simulink model "poster2"  (R2022a)
settings: Solver=VariableStepAuto  StartTime=0.0  StopTime=10.0  RelTol=1e-3
settings Model: Creator=feyzi  LastModifiedBy=feyzi

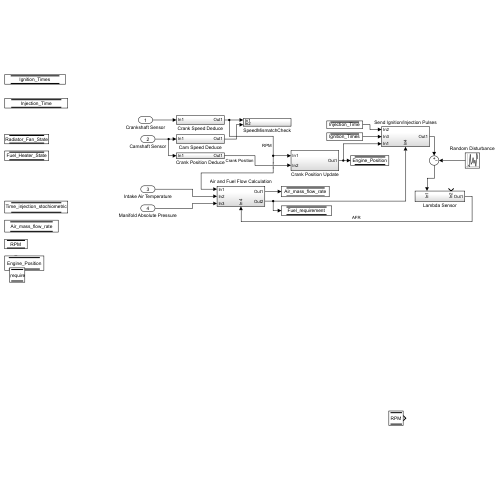
[thumbnail: Simulink's stored preview of the top-level diagram]
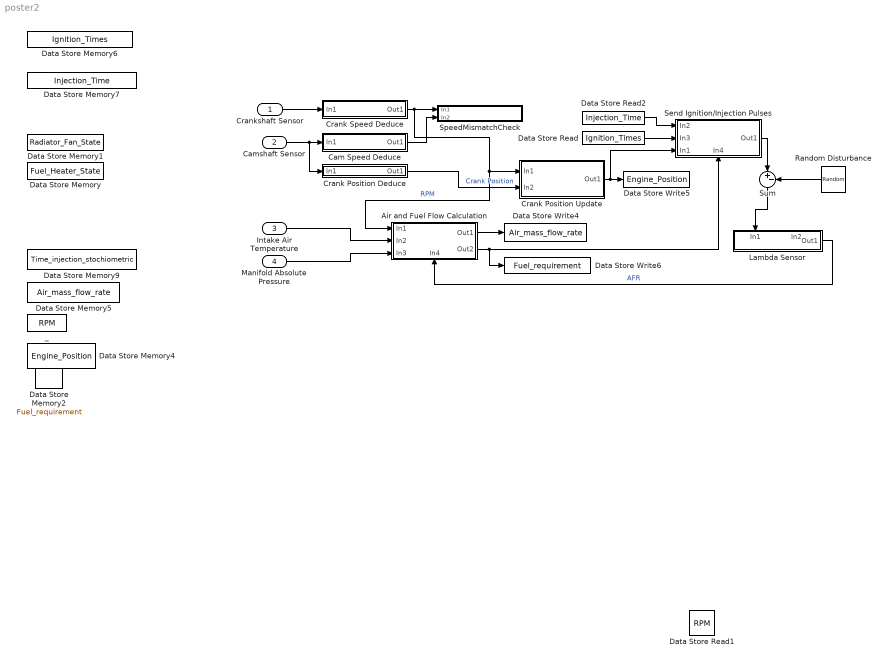
== system poster2 ==
  Crankshaft Sensor : Inport
  Camshaft Sensor : Inport  Port=2
  Intake Air Temperature : Inport  Port=3
  Manifold Absolute Pressure : Inport  Port=4
  Air and Fuel Flow Calculation : Subsystem
      settings: PortSchema="{\"entries\":[{\"content\":{\"sides\":[{\"content\":{\"connectorIds\":[\"In1\",\"In2\",\"In3\"]},\"type\":\"ConnectorPlacement.EquallySpacedRectSide\",\"uuid\":\"1a80d675-76df-4a65-b0a2-1f1f980be6c0\"},{\"content\":{\"connectorIds\":[\"Out1\",\"Out2\"],\"side\":\"RIGHT\"},\"type\":\"ConnectorPlacement.EquallySpacedRectSide\",\"uuid\":\"8955b592-f731-49d0-95be-21f996fa39e2\"},{\"content\":{\"connectorIds\":[],\"side\":\"TOP\"},\"type\":\"ConnectorPlacement.EquallySpacedRectSide\",\"uuid\":\"17a49bf9-f9ef-40a2-97c4-5293cd0c2b79\"},{\"content\":{\"connectorIds\":[\"In4\"],\"side\":\"BOTTOM\"},\"type\":\"ConnectorPlacement.EquallySpacedRectSide\",\"uuid\":\"0b8d33c3-a573-49dc-98b4-2c523fb61e9a\"}]},\"type\":\"ConnectorPlacement.EquallySpacedConnector\",\"uuid\":\"260580cd-7983-4c41-a340-dd72d4798db4\"}],\"packageUris\":[\"http://schema.mathworks.com/mf0/Connector/R2020b\"],\"version\":\"1.0\"}"
  Cam Speed Deduce : Subsystem
  Crank Position Deduce : Subsystem
  Crank Position Update : Subsystem
  Crank Speed Deduce : Subsystem
  Data Store Memory : DataStoreMemory  DataStoreName=Fuel_Heater_State  WriteAfterWriteMsg=warning  ShowAdditionalParam=off
  Data Store Memory1 : DataStoreMemory  DataStoreName=Radiator_Fan_State  WriteAfterWriteMsg=warning  ShowAdditionalParam=off
  Data Store Memory2 : DataStoreMemory  DataStoreName=Fuel_requirement  WriteAfterWriteMsg=warning  ShowAdditionalParam=off
  Data Store Memory4 : DataStoreMemory  DataStoreName=Engine_Position  WriteAfterWriteMsg=warning  ShowAdditionalParam=off
  Data Store Memory5 : DataStoreMemory  DataStoreName=Air_mass_flow_rate  WriteAfterWriteMsg=warning  ShowAdditionalParam=off
  Data Store Memory6 : DataStoreMemory  DataStoreName=Ignition_Times  WriteAfterWriteMsg=warning  ShowAdditionalParam=off
  Data Store Memory7 : DataStoreMemory  DataStoreName=Injection_Time  WriteAfterWriteMsg=warning  ShowAdditionalParam=off
  Data Store Memory9 : DataStoreMemory  DataStoreName=Time_injection_stochiometric  WriteAfterWriteMsg=warning  ShowAdditionalParam=off
  Data Store Read : DataStoreRead  DataStoreName=Ignition_Times  IndexOptions=Index vector (dialog)  Indices=1  OutputSizes=1
  Data Store Read1 : DataStoreRead  DataStoreName=RPM  IndexOptions=Index vector (dialog)  Indices=1  OutputSizes=1
  Data Store Read2 : DataStoreRead  DataStoreName=Injection_Time  IndexOptions=Index vector (dialog)  Indices=1  OutputSizes=1
  Data Store Write4 : DataStoreWrite  DataStoreName=Air_mass_flow_rate  IndexOptions=Index vector (dialog)  Indices=1  OutputSizes=1
  Data Store Write5 : DataStoreWrite  DataStoreName=Engine_Position  IndexOptions=Index vector (dialog)  Indices=1  OutputSizes=1
  Data Store Write6 : DataStoreWrite  DataStoreName=Fuel_requirement  IndexOptions=Index vector (dialog)  Indices=1  OutputSizes=1
  Lambda Sensor : Subsystem
      settings: PortSchema="{\"entries\":[{\"content\":{\"sides\":[{\"content\":{\"connectorIds\":[]},\"type\":\"ConnectorPlacement.EquallySpacedRectSide\",\"uuid\":\"be7673b4-920b-4ebb-aa7f-ea6b5173dfc7\"},{\"content\":{\"connectorIds\":[\"Out1\"],\"side\":\"RIGHT\"},\"type\":\"ConnectorPlacement.EquallySpacedRectSide\",\"uuid\":\"a4fdee98-027b-48e3-870e-bdd43bb26549\"},{\"content\":{\"connectorIds\":[\"In1\",\"In2\"],\"side\":\"TOP\"},\"type\":\"ConnectorPlacement.EquallySpacedRectSide\",\"uuid\":\"3b229d74-d616-4c69-9b14-1ea4c4b65dd7\"}]},\"type\":\"ConnectorPlacement.EquallySpacedConnector\",\"uuid\":\"497facf7-9108-426d-a3a1-d613d467dcb2\"}],\"packageUris\":[\"http://schema.mathworks.com/mf0/Connector/R2020b\"],\"version\":\"1.0\"}"
  Random Disturbance : UniformRandomNumber  SampleTime=0.1
  Send Ignition/Injection Pulses : Subsystem
      settings: PortSchema="{\"entries\":[{\"content\":{\"sides\":[{\"content\":{\"connectorIds\":[\"In1\",\"In2\",\"In3\"]},\"type\":\"ConnectorPlacement.EquallySpacedRectSide\",\"uuid\":\"1a80d675-76df-4a65-b0a2-1f1f980be6c0\"},{\"content\":{\"connectorIds\":[\"Out1\"],\"side\":\"RIGHT\"},\"type\":\"ConnectorPlacement.EquallySpacedRectSide\",\"uuid\":\"8955b592-f731-49d0-95be-21f996fa39e2\"},{\"content\":{\"connectorIds\":[],\"side\":\"TOP\"},\"type\":\"ConnectorPlacement.EquallySpacedRectSide\",\"uuid\":\"17a49bf9-f9ef-40a2-97c4-5293cd0c2b79\"},{\"content\":{\"connectorIds\":[\"In4\"],\"side\":\"BOTTOM\"},\"type\":\"ConnectorPlacement.EquallySpacedRectSide\",\"uuid\":\"08643730-c224-4892-94d3-b722ab0d9115\"}]},\"type\":\"ConnectorPlacement.EquallySpacedConnector\",\"uuid\":\"260580cd-7983-4c41-a340-dd72d4798db4\"}],\"packageUris\":[\"http://schema.mathworks.com/mf0/Connector/R2020b\"],\"version\":\"1.0\"}"
  SpeedMismatchCheck : Subsystem
  Sum : Sum  Inputs=|+-
  _ : DataStoreMemory  DataStoreName=RPM  WriteAfterWriteMsg=warning  ShowAdditionalParam=off
  wires:
  Data Store Read2/1 -> Send Ignition/Injection Pulses/1(In2)
  Random Disturbance/1 -> Sum/2
  Crank Position Update/1(Out1) -> Send Ignition/Injection Pulses/3(In1), Data Store Write5/1
  Manifold Absolute Pressure/1 -> Air and Fuel Flow Calculation/3(In3)
  Air and Fuel Flow Calculation/1(Out1) -> Data Store Write4/1
  Intake Air Temperature/1 -> Air and Fuel Flow Calculation/2(In2)
  Lambda Sensor/1(Out1) -> Air and Fuel Flow Calculation/4(In4)  "AFR"
  Data Store Read/1 -> Send Ignition/Injection Pulses/2(In3)
  Crank Position Deduce/1(Out1) -> Crank Position Update/2(In2)  "Crank Position"
  Cam Speed Deduce/1(Out1) -> SpeedMismatchCheck/2(In2)
  Crankshaft Sensor/1 -> Crank Speed Deduce/1(In1)
  Camshaft Sensor/1 -> Cam Speed Deduce/1(In1), Crank Position Deduce/1(In1)
  Air and Fuel Flow Calculation/2(Out2) -> Data Store Write6/1, Send Ignition/Injection Pulses/4(In4)
  Crank Speed Deduce/1(Out1) -> Air and Fuel Flow Calculation/1(In1), Crank Position Update/1(In1), SpeedMismatchCheck/1(In1)  "RPM"
  Send Ignition/Injection Pulses/1(Out1) -> Sum/1
  Sum/1 -> Lambda Sensor/1(In1)

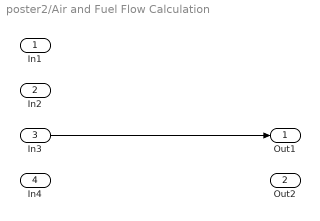
== system poster2/Air and Fuel Flow Calculation ==
  In1 : Inport
  In2 : Inport  Port=2
  In3 : Inport  Port=3
  In4 : Inport  Port=4
  Out1 : Outport
  Out2 : Outport  Port=2
  wires:
  In3/1 -> Out1/1

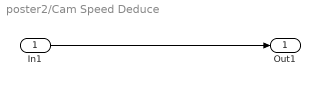
== system poster2/Cam Speed Deduce ==
  In1 : Inport
  Out1 : Outport
  wires:
  In1/1 -> Out1/1

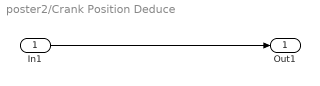
== system poster2/Crank Position Deduce ==
  In1 : Inport
  Out1 : Outport
  wires:
  In1/1 -> Out1/1

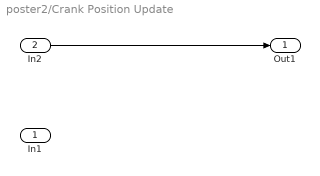
== system poster2/Crank Position Update ==
  In1 : Inport
  In2 : Inport  Port=2
  Out1 : Outport
  wires:
  In2/1 -> Out1/1

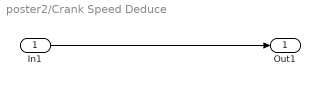
== system poster2/Crank Speed Deduce ==
  In1 : Inport
  Out1 : Outport
  wires:
  In1/1 -> Out1/1

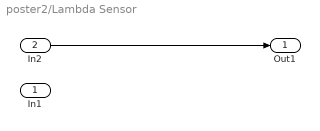
== system poster2/Lambda Sensor ==
  In1 : Inport
  In2 : Inport  Port=2
  Out1 : Outport
  wires:
  In2/1 -> Out1/1

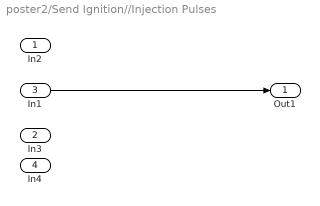
== system poster2/Send Ignition//Injection Pulses ==
  In2 : Inport
  In3 : Inport  Port=2
  In1 : Inport  Port=3
  In4 : Inport  Port=4
  Out1 : Outport
  wires:
  In1/1 -> Out1/1

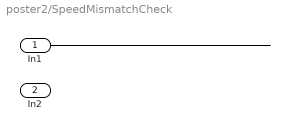
== system poster2/SpeedMismatchCheck ==
  In1 : Inport
  In2 : Inport  Port=2
  wires:
  In1/1 -> ?
